simulink model "Target_Control_System"  (R2021b)
settings: Solver=FixedStepDiscrete  StartTime=0.0  StopTime=5  RelTol=1e-3
PreLoadFcn:
  | RTWConfigurationCB('preloadfcn', bdroot);
PostLoadFcn:
  | load('configuration/data_struct.mat');
  | load('configuration/fluxMaps_propMotor.mat');
  | load('configuration/parameterInit_PROP.mat');
  | load('configuration/parameterInit_PUMP.mat');
  | load('configuration/parameterInit_PITCH.mat');
  | load('configuration/parameterInit_TILT.mat');
  | %load('configuration/base_workspace_signal_definition.mat');
  | %load('resolvedatastores_to_baseworkspace_for_faster_simulation.mat');
model workspace (MAT data in the model file):
  SIMULATION_OPTIONS : Simulink.Parameter (value not decoded)
  TARGET_CODE_GEN : Simulink.Parameter (value not decoded)
  TCS_SAMPLE_FREQ_HZ : Simulink.Parameter (value not decoded)
symbols that are objects in the model workspace (value not decoded): TARGET_CODE_GEN, TCS_SAMPLE_FREQ_HZ
undefined symbols (not defined in the file): A_DQ_REF_LPF_INIT__PITCH, A_DQ_REF_LPF_INIT__PROP, A_DQ_REF_LPF_INIT__PUMP, A_DQ_REF_LPF_INIT__TILT, A_OBSERVER_CONFIDENCE_INIT__PITCH, A_OBSERVER_CONFIDENCE_INIT__PROP, A_OBSERVER_CONFIDENCE_INIT__PUMP, A_OBSERVER_CONFIDENCE_INIT__TILT, ACTUATOR_MAX_ANGLE_TRIP__PITCH, ACTUATOR_MIN_ANGLE_TRIP__PITCH, ACTUATOR_POS_SENSOR_INV_DIRECTION__PITCH, ACTUATOR_POS_SENSOR_INV_DIRECTION__TILT, ACTUATOR_POS_SENSOR_OFFSET__PITCH, ACTUATOR_POS_SENSOR_OFFSET__TILT, ADC_scaler1_baseaddr_TILT, ADC_SCALER_FLOAT_TO_FIXPOINT_EXPANSION, ANGLE_ELEC_FROM_SENSOR_OFFSET_INIT__PITCH, ANGLE_ELEC_FROM_SENSOR_OFFSET_INIT__PROP, ANGLE_ELEC_FROM_SENSOR_OFFSET_INIT__PUMP, ANGLE_ELEC_FROM_SENSOR_OFFSET_INIT__TILT, AUTO_CLEAR_FAULTS_ENABLED__PITCH, AUTO_CLEAR_FAULTS_ENABLED__PROP, AUTO_CLEAR_FAULTS_ENABLED__PUMP, AUTO_CLEAR_FAULTS_ENABLED__TILT, AUTO_CLEAR_FAULTS_WAIT_TICKS__PITCH, AUTO_CLEAR_FAULTS_WAIT_TICKS__PROP, AUTO_CLEAR_FAULTS_WAIT_TICKS__PUMP, AUTO_CLEAR_FAULTS_WAIT_TICKS__TILT, AUTO_I_ZERO_IDLE_TICKS__PITCH, AUTO_I_ZERO_IDLE_TICKS__PROP, AUTO_I_ZERO_IDLE_TICKS__PUMP, AUTO_I_ZERO_IDLE_TICKS__TILT, AUTO_I_ZERO_OFFSET_IDC_THRESHOLD__PITCH, AUTO_I_ZERO_OFFSET_IDC_THRESHOLD__PROP, AUTO_I_ZERO_OFFSET_IDC_THRESHOLD__PUMP, AUTO_I_ZERO_OFFSET_IDC_THRESHOLD__TILT, AUTO_I_ZERO_OFFSET_IPH_THRESHOLD__PITCH, AUTO_I_ZERO_OFFSET_IPH_THRESHOLD__PROP, AUTO_I_ZERO_OFFSET_IPH_THRESHOLD__PUMP, AUTO_I_ZERO_OFFSET_IPH_THRESHOLD__TILT, AUTO_SENSORLESS_SWITCHOVER_DISABLE_OMEGA, AUTO_SENSORLESS_SWITCHOVER_ENABLE_OMEGA, AUTO_SENSORLESS_SWITCHOVER_MIN_CONFIDENCE, AUXILIARY_PROTECTION_UNIT_BASEADDR__TILT, blanking_max_error_omega_INIT_PITCH, blanking_max_error_omega_INIT_TILT, blanking_max_error_position_INIT_PITCH, blanking_max_error_position_INIT_TILT, BRUTE_START_I_Q_REF_RAMP_SPEED__PITCH, BRUTE_START_I_Q_REF_RAMP_SPEED__PROP, BRUTE_START_I_Q_REF_RAMP_SPEED__PUMP, BRUTE_START_I_Q_REF_RAMP_SPEED__TILT, CONTROL_LOOP_DT_INIT__PITCH, CONTROL_LOOP_DT_INIT__PROP, CONTROL_LOOP_DT_INIT__PUMP, CONTROL_LOOP_DT_INIT__TILT, CORRECTION_FILTER_SCALE__PITCH, CORRECTION_FILTER_SCALE__PROP, CORRECTION_FILTER_SCALE__PUMP, CORRECTION_FILTER_SCALE__TILT ... (+458)
libraries: simulink x178, Reusables_Lib x24
(part 13 of 47)

== system Target_Control_System/Target_Control_System/InterruptFunction/tiltMotor_isrTask/pwmGeneration/Subsystem ==
  Enable : EnablePort
  ABC to DQ : Subsystem
  Calculate Duty Cycles : Subsystem
  Constant : Constant  OutDataTypeStr=int32  SampleTime=-1
  Constant1 : Constant  Commented=on  OutDataTypeStr=uint32  SampleTime=-1
  Data Store Read1 : DataStoreRead  DataStoreName=mdl_tilt_fFluxMasterAngleBkwd_cos_  IndexOptions=Index vector (dialog)  Indices=1  OutputSizes=1
  Data Store Read13 : DataStoreRead  DataStoreName=mdl_tilt_fFluxMasterAngleBkwd_sin_  IndexOptions=Index vector (dialog)  Indices=1  OutputSizes=1
  Data Store Read2 : DataStoreRead  DataStoreName=oTilt  DataStoreElements=oTilt.oIsr_.oParam_.iInverseDirection_  IndexOptions=Index vector (dialog)  Indices=1  OutputSizes=1
  Data Store Read3 : DataStoreRead  DataStoreName=oTilt  DataStoreElements=oTilt.oIsr_.oState_.fUdRef_  IndexOptions=Index vector (dialog)  Indices=1  OutputSizes=1
  Data Store Read4 : DataStoreRead  DataStoreName=oTilt  DataStoreElements=oTilt.oIsr_.oState_.fUqRef_  IndexOptions=Index vector (dialog)  Indices=1  OutputSizes=1
  Data Store Read6 : DataStoreRead  DataStoreName=oTilt  DataStoreElements=oTilt.oIsr_.oParam_.fMaximumDuty_  IndexOptions=Index vector (dialog)  Indices=1  OutputSizes=1
  Data Store Read7 : DataStoreRead  DataStoreName=oTilt  DataStoreElements=oTilt.oIsr_.oParam_.fHalfPositiveDuty_  IndexOptions=Index vector (dialog)  Indices=1  OutputSizes=1
  Data Store Read8 : DataStoreRead  DataStoreName=oTilt  DataStoreElements=oTilt.oIsr_.oParam_.fPwmPeriodTicksFloat_  IndexOptions=Index vector (dialog)  Indices=1  OutputSizes=1
  Data Store Write : DataStoreWrite  DataStoreName=oTilt  DataStoreElements=oTilt.oIsr_.oOut_.uiPwmDutyTicksA_  IndexOptions=Index vector (dialog)  Indices=1  OutputSizes=1
  Data Store Write1 : DataStoreWrite  DataStoreName=oTilt  DataStoreElements=oTilt.oIsr_.oOut_.uiPwmDutyTicksB_  IndexOptions=Index vector (dialog)  Indices=1  OutputSizes=1
  Data Store Write2 : DataStoreWrite  DataStoreName=oTilt  DataStoreElements=oTilt.oIsr_.oOut_.uiPwmDutyTicksC_  IndexOptions=Index vector (dialog)  Indices=1  OutputSizes=1
  Data Store Write3 : DataStoreWrite  Commented=on  DataStoreName=oTilt  DataStoreElements=oTilt.oIsr_.oOut_.uiPwmSetByIsr_  IndexOptions=Index vector (dialog)  Indices=1  OutputSizes=1
  Data Store Write4 : DataStoreWrite  DataStoreName=oTilt  DataStoreElements=oTilt.oIsr_.oState_.iPwmUpdated_  IndexOptions=Index vector (dialog)  Indices=1  OutputSizes=1
  Zero sequence injection : Subsystem
  wires:
  Constant1/1 -> Data Store Write3/1
  Data Store Read1/1 -> ABC to DQ/5(fFluxMasterAngleBkwd_cos)
  Data Store Read13/1 -> ABC to DQ/4(fFluxMasterAngleBkwd_sin)
  Calculate Duty Cycles/3(uiPwmDutyTicksC) -> Data Store Write2/1
  Calculate Duty Cycles/2(uiPwmDutyTicksB) -> Data Store Write1/1
  Calculate Duty Cycles/1(uiPwmDutyTicksA) -> Data Store Write/1
  Data Store Read3/1 -> ABC to DQ/2(UdRef)
  Data Store Read4/1 -> ABC to DQ/3(UqRef)
  Data Store Read8/1 -> Calculate Duty Cycles/6(fPwmPeriodTicksFloat)
  Data Store Read7/1 -> Calculate Duty Cycles/5(fHalfPositiveDuty)
  Data Store Read6/1 -> Calculate Duty Cycles/4(fMaximumDuty)
  Data Store Read2/1 -> ABC to DQ/1(iInverseDirection)
  Zero sequence injection/3(fUcRef) -> Calculate Duty Cycles/3(fUcRef)
  Zero sequence injection/2(fUbRef) -> Calculate Duty Cycles/2(fUbRef)
  Zero sequence injection/1(fUaRef) -> Calculate Duty Cycles/1(fUaRef)
  ABC to DQ/1(U_abc) -> Zero sequence injection/1(U_abc)
  Constant/1 -> Data Store Write4/1

== system Target_Control_System/Target_Control_System/InterruptFunction/tiltMotor_setPwm/ModelSourceFPGATilt/DoNotIncludeCustomCode ==

== system Target_Control_System/Target_Control_System/InterruptFunction/tiltMotor_setPwm/ModelSourceFPGATilt/IncludeCustomCode ==
  System Update : Subsystem  mask(System Update){ShowInLibBrowser=0}
      mask prompts: ShowInLibBrowser "Simulink:masks:CustCodeMaskParam1_MP"
      settings: CopyFcn=cccopyfcn(gcb)  OpenFcn=ccopenfcn('System Update Function')
      mask Help: eval('feval(''rtwprivate'',''rtwhelpview'',''rtw_sys_update_block'')');
      mask DialogControl ShowInLibBrowser Prompt: Mask Parameter 1:
      mask Display: disp('System\nUpdate');

== system Target_Control_System/Target_Control_System/MainLoop/pitchMotor_mainLoop/Decimation gate for 10 Hz Pitch/Function-Call Subsystem ==
  motorTaskMainDecimationBStep_pitch : TriggerPort  TriggerType=function-call  VariantControl=Variant
  DC_overvoltage_pitch : Stateflow chart  TreatAsAtomicUnit=on
  Dynamic_current_limiting_pitch : Subsystem

== system Target_Control_System/Target_Control_System/MainLoop/pitchMotor_mainLoop/Decimation gate for 200 Hz Pitch/Function-Call Subsystem ==
  motorTaskMainDecimationAStep_pitch : TriggerPort  TriggerType=function-call  VariantControl=Variant
  Check zero current if inverter off : Subsystem  TreatAsAtomicUnit=on
  Current control inactive : Subsystem  TreatAsAtomicUnit=on
  Current offset nulling : Subsystem  TreatAsAtomicUnit=on
  DClink_overCurrentProtection : Subsystem  TreatAsAtomicUnit=on
  Forced current injection for broken input sensors : Subsystem  Commented=on  TreatAsAtomicUnit=on
  Function-Call Generator : simulink/Ports & Subsystems/Function-Call Generator  sample_time=-1  numberOfIterations=1  DisallowWideOutput=off
  Function-Call Split{1..5,10} (6 alike) : FunctionCallSplit  NumOutputPorts=2
  Idle controller : Subsystem  TreatAsAtomicUnit=on
  Position control checks : Subsystem  TreatAsAtomicUnit=on
  wires:
  Function-Call Split10/2 -> Function-Call Split1/1
  Function-Call Split3/2 -> Function-Call Split4/1
  Function-Call Generator/1 -> Function-Call Split10/1
  Function-Call Split3/1 -> Current control inactive/Trigger
  Function-Call Split1/1 -> Check zero current if inverter off/Trigger
  Function-Call Split10/1 -> DClink_overCurrentProtection/Trigger
  Function-Call Split2/2 -> Function-Call Split3/1
  Function-Call Split5/1 -> Idle controller/Trigger
  Function-Call Split1/2 -> Function-Call Split2/1
  Function-Call Split4/1 -> Forced current injection for broken input sensors/Trigger
  Function-Call Split2/1 -> Current offset nulling/Trigger
  Function-Call Split5/2 -> Position control checks/Trigger
  Function-Call Split4/2 -> Function-Call Split5/1

== system Target_Control_System/Target_Control_System/MainLoop/pitchMotor_mainLoop/Decimation gate for 5000 Hz Pitch/motorTaskProcessExternalSetpoints(&oPitch) ==
  note: // Do not set certain variables during auto forced angle start or resistance measurement // This whole code below should be cleaned up, probably a switch case tied to the state machine.
      | // The different modes, (position control, speed control, current control) should get different state numbers to facilitate this.
  note: // Take externally requested setpoints (already set in the 'in' struct) and apply them (after sanitizing) to the right place in the control loop, also depending on the state that the drive is in.
  motorTaskProcessExternalSetpoints : TriggerPort  TriggerType=function-call  VariantControl=Variant
  Function-Call Generator : simulink/Ports & Subsystems/Function-Call Generator  sample_time=-1  numberOfIterations=1  DisallowWideOutput=off
  Function-Call Split1 : FunctionCallSplit  NumOutputPorts=2
  Function-Call Split10 : FunctionCallSplit  NumOutputPorts=2
  hot_standby : Subsystem
  passive_holding_mode : Subsystem
  set_target : Subsystem
  wires:
  Function-Call Split1/2 -> set_target/Trigger
  Function-Call Split10/2 -> Function-Call Split1/1
  Function-Call Split1/1 -> hot_standby/Trigger
  Function-Call Split10/1 -> passive_holding_mode/Trigger
  Function-Call Generator/1 -> Function-Call Split10/1

== system Target_Control_System/Target_Control_System/MainLoop/pitchMotor_mainLoop/mainTask_pitch/PWM for Simulation ==
  Enable : EnablePort
  Bus Creator3 : BusCreator  Inputs=3
  Constant : Constant  OutDataTypeStr=uint32  SampleTime=-1
  Constant{1..4} (4 alike) : Constant  Value=0  OutDataTypeStr=uint32  SampleTime=-1
  Data Store Read1 : DataStoreRead  DataStoreName=oPitch  DataStoreElements=oPitch.oIsr_.oState_.iPwmUpdated_  IndexOptions=Index vector (dialog)  Indices=1  OutputSizes=1
  Data Store Read9 : DataStoreRead  DataStoreName=oPitch  DataStoreElements=oPitch.oMot_.oOut_.uiEnableGateDrive_  IndexOptions=Index vector (dialog)  Indices=1  OutputSizes=1
  Data Store Write18 : DataStoreWrite  DataStoreName=oPitch  DataStoreElements=oPitch.oIsr_.oOut_.uiPwmSetByIsr_  IndexOptions=Index vector (dialog)  Indices=1  OutputSizes=1
  NOT : Logic  Operator=NOT  AllPortsSameDT=off  OutDataTypeStr=boolean
  Scope : Scope
  Subsystem : Subsystem
  Subsystem1 : Subsystem
  Switch1 : Switch  Criteria=u2 > Threshold
  Switch2 : Switch  Criteria=u2 > Threshold
  Switch3 : Switch  Criteria=u2 > Threshold
  Out1 : Outport
  wires:
  Switch3/1 -> Data Store Write18/1
  Constant4/1 -> Switch3/3
  Subsystem/1(pitchMotor_PWMticks) -> Switch2/1
  Constant/1 -> Switch3/1
  Subsystem1/1(pitchMotor_PWMticks) -> Switch2/3
  Data Store Read1/1 -> Subsystem/Enable, Switch2/2, NOT/1, Scope/1, Switch3/2
  NOT/1 -> Subsystem1/Enable
  Data Store Read9/1 -> Switch1/2
  Switch2/1 -> Switch1/1  "pitchMotor_PWMticks"
  Constant1/1 -> Bus Creator3/1  "Aticks"
  Constant2/1 -> Bus Creator3/2  "Bticks"
  Switch1/1 -> Out1/1  "pitchMotor_PWMticks"
  Constant3/1 -> Bus Creator3/3  "Cticks"
  Bus Creator3/1 -> Switch1/3

== system Target_Control_System/Target_Control_System/MainLoop/pitchMotor_mainLoop/mainTask_pitch/Variant Subsystem ==
  note: 1) Add Subsystem or Model blocks as valid variant choices.
      | 2) You cannot connect blocks at this level. At simulation, connectivity is automatically
      | determined, based on the active variant and port name matching.
  Target_Code_Gen_0 : Subsystem  VariantControl=(default)
  Target_Code_Gen_1 : Subsystem  VariantControl=TARGET_CODE_GEN==1
  Output : Outport  OutputFunctionCall=on

== system Target_Control_System/Target_Control_System/MainLoop/pitchMotor_mainLoop/mainTask_pitch/motorTaskMainFastStep() ==
  motorTaskMainFastStep : TriggerPort  TriggerType=function-call  VariantControl=Variant
  Automatic switching to sensorless - Pitch : Subsystem  Commented=on
  Control Loops - Pitch : Subsystem
  Correction Constants for Observer and Control - Pitch : Subsystem  Commented=on
  Function-Call Generator : simulink/Ports & Subsystems/Function-Call Generator  sample_time=-1  numberOfIterations=1  DisallowWideOutput=off
  Function-Call Split{1..6,10} (7 alike) : FunctionCallSplit  NumOutputPorts=2
  Lowpass Filtered Quantities for External World - Pitch : Subsystem
  Mechanical System - Pitch : Subsystem
  Motor Acceleration - Pitch : Subsystem
  Observer Confidence - Pitch : Subsystem  Commented=on
  Software Overcurrent Protection - Pitch : Subsystem
  enableDrive(&oPitch) : Stateflow chart  TreatAsAtomicUnit=on
  initiateOffsetNulling(&oPitch) : Stateflow chart  TreatAsAtomicUnit=on
  wires:
  Function-Call Split6/2 -> Motor Acceleration - Pitch/Trigger
  Function-Call Split6/1 -> Correction Constants for Observer and Control - Pitch/Trigger
  Function-Call Split5/2 -> Function-Call Split6/1
  Function-Call Split5/1 -> Control Loops - Pitch/Trigger
  Function-Call Split4/2 -> Function-Call Split5/1
  Function-Call Split4/1 -> Lowpass Filtered Quantities for External World - Pitch/Trigger
  Function-Call Split3/2 -> Function-Call Split4/1
  Function-Call Split3/1 -> Automatic switching to sensorless - Pitch/Trigger
  Function-Call Split2/2 -> Function-Call Split3/1
  Function-Call Split2/1 -> Observer Confidence - Pitch/Trigger
  Function-Call Split1/2 -> Function-Call Split2/1
  Function-Call Split1/1 -> Mechanical System - Pitch/Trigger
  Function-Call Generator/1 -> Function-Call Split10/1
  Function-Call Split10/1 -> Software Overcurrent Protection - Pitch/Trigger
  Function-Call Split10/2 -> Function-Call Split1/1

== system Target_Control_System/Target_Control_System/MainLoop/pitchMotor_mainLoop/mainTask_pitch/motorTaskManagePwmRequestFlags() ==
  motorTaskManagePwmRequestFlags : TriggerPort  TriggerType=function-call  VariantControl=Variant
  Constant : Constant  Value=0  OutDataTypeStr=uint32  SampleTime=-1
  Data Store Read : DataStoreRead  DataStoreName=oPitch  DataStoreElements=oPitch.oMot_.oIn_.uiPwmSetByIsr_  IndexOptions=Index vector (dialog)  Indices=1  OutputSizes=1
  Data Store Read1 : DataStoreRead  DataStoreName=oPitch  DataStoreElements=oPitch.oMot_.oOut_.uiPwmRequestFromMain_  IndexOptions=Index vector (dialog)  Indices=1  OutputSizes=1
  Data Store Write : DataStoreWrite  DataStoreName=oPitch  DataStoreElements=oPitch.oMot_.oOut_.uiPwmRequestFromMain_  IndexOptions=Index vector (dialog)  Indices=1  OutputSizes=1
  Switch : Switch  Criteria=u2 > Threshold  OutDataTypeStr=uint32
  wires:
  Data Store Read1/1 -> Switch/3
  Constant/1 -> Switch/1
  Switch/1 -> Data Store Write/1
  Data Store Read/1 -> Switch/2

== system Target_Control_System/Target_Control_System/MainLoop/pitchMotor_mainLoop/mainTask_pitch/resetFlag_uiDataFromIsrToMainUpdated ==
  resetFlag_uiDataFromIsrToMainUpdated : TriggerPort  TriggerType=function-call  VariantControl=Variant
  Constant : Constant  Value=0  OutDataTypeStr=uint32  SampleTime=-1
  Data Store Write : DataStoreWrite  DataStoreName=oPitch  DataStoreElements=oPitch.oMot_.oIn_.uiDataFromIsrToMainUpdated_  IndexOptions=Index vector (dialog)  Indices=1  OutputSizes=1
  wires:
  Constant/1 -> Data Store Write/1

== system Target_Control_System/Target_Control_System/MainLoop/propMotor_mainLoop/Decimation gate A for 200 Hz Prop/Cross-tripping VP//Tilt to Prop ==
  Tilt to Prop : Stateflow chart  TreatAsAtomicUnit=on
  VP to Prop : Stateflow chart  TreatAsAtomicUnit=on

== system Target_Control_System/Target_Control_System/MainLoop/propMotor_mainLoop/Decimation gate A for 200 Hz Prop/Current offset nulling ==
  note: Try to perform current sensor offset nulling at least once as soon as possible:
      | (Subsequent nulling steps are performed only once the drive has been idle for a while)
  function : TriggerPort  TriggerType=function-call  VariantControl=Variant
  Constant2 : Constant  Value=0  OutDataTypeStr=uint32  SampleTime=-1
  Data Store Read2 : DataStoreRead  DataStoreName=oProp  DataStoreElements=oProp.oMot_.oState_.uiCurrentOffsetNullingPerformed_  IndexOptions=Index vector (dialog)  Indices=1  OutputSizes=1
  GreaterThan1 : RelationalOperator  Operator=>  OutDataTypeStr=boolean  RndMeth=Simplest
  NOT : Logic  Operator=NOT  IconShape=distinctive  AllPortsSameDT=off  OutDataTypeStr=boolean
  initiateOffsetNulling(&oProp) : Subsystem  TreatAsAtomicUnit=on
  wires:
  NOT/1 -> initiateOffsetNulling(&oProp)/Enable
  GreaterThan1/1 -> NOT/1
  Constant2/1 -> GreaterThan1/2
  Data Store Read2/1 -> GreaterThan1/1

== system Target_Control_System/Target_Control_System/MainLoop/propMotor_mainLoop/Decimation gate A for 200 Hz Prop/Subsystem ==
  Idle_Controller : TriggerPort  TriggerType=function-call  VariantControl=Variant
  AND7 : Logic  AllPortsSameDT=off  OutDataTypeStr=boolean
  Data Store Read1 : DataStoreRead  DataStoreName=oProp  DataStoreElements=oProp.oMot_.oParam_.oPiDataIdleCtrl_.fState_  IndexOptions=Index vector (dialog)  Indices=1  OutputSizes=1
  Data Store Read12 : DataStoreRead  DataStoreName=oProp  DataStoreElements=oProp.oMot_.oState_.uiDriveState_  IndexOptions=Index vector (dialog)  Indices=1  OutputSizes=1
  Data Store Read2 : DataStoreRead  DataStoreName=oProp  DataStoreElements=oProp.oMot_.oParam_.fRpmBlankingUnblankConfidence_  IndexOptions=Index vector (dialog)  Indices=1  OutputSizes=1
  Data Store Read3 : DataStoreRead  DataStoreName=oProp  DataStoreElements=oProp.oMot_.oParam_.fRpmBlankingBlankConfidence_  IndexOptions=Index vector (dialog)  Indices=1  OutputSizes=1
  Data Store Read51 : DataStoreRead  DataStoreName=oProp  DataStoreElements=oProp.oMot_.oState_.uiDriveState_  IndexOptions=Index vector (dialog)  Indices=1  OutputSizes=1
  Data Store Read65 : DataStoreRead  DataStoreName=oProp  DataStoreElements=oProp.oMot_.oOut_.fOmegaEObserverXlpf2_  IndexOptions=Index vector (dialog)  Indices=1  OutputSizes=1
  Data Store Read66 : DataStoreRead  DataStoreName=oProp  DataStoreElements=oProp.oMot_.oState_.fIdleCtrlOmegaEMin_  IndexOptions=Index vector (dialog)  Indices=1  OutputSizes=1
  Data Store Read67 : DataStoreRead  DataStoreName=oProp  DataStoreElements=oProp.oMot_.oParam_.oPiDataIdleCtrl_.oParameter_.fKp_  IndexOptions=Index vector (dialog)  Indices=1  OutputSizes=1
  Data Store Read69 : DataStoreRead  DataStoreName=oProp  DataStoreElements=oProp.oMot_.oParam_.oPiDataIdleCtrl_.oParameter_.fKi_  IndexOptions=Index vector (dialog)  Indices=1  OutputSizes=1
  Data Store Read70 : DataStoreRead  DataStoreName=oProp  DataStoreElements=oProp.oMot_.oParam_.oPiDataIdleCtrl_.oParameter_.fIntMax_  IndexOptions=Index vector (dialog)  Indices=1  OutputSizes=1
  Data Store Read80 : DataStoreRead  DataStoreName=oProp  DataStoreElements=oProp.oMot_.oState_.fObserverConfidence_  IndexOptions=Index vector (dialog)  Indices=1  OutputSizes=1
  Data Store Read94 : DataStoreRead  DataStoreName=oProp  DataStoreElements=oProp.oMot_.oParam_.oPiDataIdleCtrl_.oParameter_.fOutMax_  IndexOptions=Index vector (dialog)  Indices=1  OutputSizes=1
  Data Store Read95 : DataStoreRead  DataStoreName=oProp  DataStoreElements=oProp.oMot_.oParam_.oPiDataIdleCtrl_.oParameter_.fLoopDt_  IndexOptions=Index vector (dialog)  Indices=1  OutputSizes=1
  Data Store Write10 : DataStoreWrite  DataStoreName=oProp  DataStoreElements=oProp.oMot_.oState_.iRpmBlankingActive_  IndexOptions=Index vector (dialog)  Indices=1  OutputSizes=1
  Equal12 : RelationalOperator  Operator===  OutDataTypeStr=boolean  RndMeth=Simplest
  Equal16 : RelationalOperator  Operator=~=  OutDataTypeStr=boolean  RndMeth=Simplest
  Equal17 : RelationalOperator  Operator=~=  OutDataTypeStr=boolean  RndMeth=Simplest
  NOT : Logic  Operator=NOT  AllPortsSameDT=off  OutDataTypeStr=boolean
  OR (Never blank in state 200)1 : Logic  Operator=OR  AllPortsSameDT=off  OutDataTypeStr=boolean
  Subsystem : Subsystem
  Switch7 : Switch  Criteria=u2 > Threshold  Threshold=0.5  OutDataTypeStr=int32
  Zero18 : Constant  Value=0  OutDataTypeStr=single  SampleTime=-1
  Zero19 : Constant  OutDataTypeStr=single  SampleTime=-1
  Zero9 : Constant  Value=0  OutDataTypeStr=single  SampleTime=-1
  const12 : Constant  Value=200  OutDataTypeStr=uint32  SampleTime=-1
  const13 : Constant  Value=211  OutDataTypeStr=uint32  SampleTime=-1
  const14 : Constant  Value=212  OutDataTypeStr=uint32  SampleTime=-1
  greater1 : RelationalOperator  Operator=>  OutDataTypeStr=boolean  RndMeth=Simplest
  piControllerStep_Idle_Controller : Subsystem  SystemSampleTime=1/200
  smaller1 : RelationalOperator  Operator=<  OutDataTypeStr=boolean  RndMeth=Simplest
  wires:
  Data Store Read80/1 -> smaller1/1, greater1/1
  OR (Never blank in state 200)1/1 -> Switch7/2
  Zero9/1 -> Switch7/1
  smaller1/1 -> Switch7/3
  Equal12/1 -> OR (Never blank in state 200)1/1
  Data Store Read12/1 -> Equal12/1
  Data Store Read3/1 -> smaller1/2
  Data Store Read2/1 -> greater1/2
  Switch7/1 -> Data Store Write10/1
  const12/1 -> Equal12/2
  greater1/1 -> OR (Never blank in state 200)1/2
  NOT/1 -> Subsystem/Enable
  Data Store Read1/1 -> piControllerStep_Idle_Controller/11(fState)
  const13/1 -> Equal16/1
  Data Store Read67/1 -> piControllerStep_Idle_Controller/3(fKp)
  Data Store Read94/1 -> piControllerStep_Idle_Controller/8(fOutMax)
  Data Store Read66/1 -> piControllerStep_Idle_Controller/2(fTarget)
  Zero19/1 -> piControllerStep_Idle_Controller/5(fScale)
  Data Store Read70/1 -> piControllerStep_Idle_Controller/7(fIntMax)
  Data Store Read95/1 -> piControllerStep_Idle_Controller/6(fLoopDt)
  Data Store Read69/1 -> piControllerStep_Idle_Controller/4(fKi)
  Data Store Read51/1 -> Equal16/2, Equal17/1
  Equal17/1 -> AND7/2
  Zero18/1 -> piControllerStep_Idle_Controller/9(fIntMin), piControllerStep_Idle_Controller/10(fOutMin)
  AND7/1 -> piControllerStep_Idle_Controller/Enable, NOT/1
  const14/1 -> Equal17/2
  Data Store Read65/1 -> piControllerStep_Idle_Controller/1(fActual)
  Equal16/1 -> AND7/1

== system Target_Control_System/Target_Control_System/MainLoop/propMotor_mainLoop/Decimation gate for 5000 Hz Prop/motorTaskProcessExternalSetpoints(&oProp) ==
  note: // Do not set certain variables during auto forced angle start or resistance measurement // This whole code below should be cleaned up, probably a switch case tied to the state machine.
      | // The different modes, (position control, speed control, current control) should get different state numbers to facilitate this.
  note: // Take externally requested setpoints (already set in the 'in' struct) and apply them (after sanitizing) to the right place in the control loop, also depending on the state that the drive is in.
  motorTaskProcessExternalSetpoints : TriggerPort  TriggerType=function-call  VariantControl=Variant
  Function-Call Generator : simulink/Ports & Subsystems/Function-Call Generator  sample_time=-1  numberOfIterations=1  DisallowWideOutput=off
  Function-Call Split1 : FunctionCallSplit  NumOutputPorts=2
  Function-Call Split10 : FunctionCallSplit  NumOutputPorts=2
  Subsystem1 : Subsystem
  Subsystem2 : Subsystem
  Subsystem3 : Subsystem
  wires:
  Function-Call Split1/2 -> Subsystem3/Trigger
  Function-Call Split10/2 -> Function-Call Split1/1
  Function-Call Split1/1 -> Subsystem2/Trigger
  Function-Call Split10/1 -> Subsystem1/Trigger
  Function-Call Generator/1 -> Function-Call Split10/1

== system Target_Control_System/Target_Control_System/MainLoop/propMotor_mainLoop/motorTaskMainFastStep(&oProp)/Control Loops - Prop ==
  note: ---------- runFluxWeakeningCurrentCalculation ------------
      | 	// This function calculates how much flux weakening current is needed to keep the modulation index below full scale.
      | 	// It uses positive numbers exclusively for ease of reading & reasoning; the calling function
      | 	// will have to include a minus sign somewhere to turn it into negative d-current.
  note: // If the speed is too low, just return zero. // This is a simple safety catch to prevent injecting d current when there should be no need for it.
  note: mdl_fIdFluxWeakeningSetpoint_
  controlLoops : TriggerPort  TriggerType=function-call  VariantControl=Variant
  AND1 : Logic  AllPortsSameDT=off  OutDataTypeStr=boolean
  Abs6 : Abs
  Add12 : Sum  Inputs=+-
  Constant3 : Constant  Value=0  OutDataTypeStr=single  SampleTime=-1
  Data Store Read1 : DataStoreRead  DataStoreName=oProp  DataStoreElements=oProp.oMot_.oState_.oRampDataFluxMstrAngFrcd2clsdSmoothn_.oParam_.fTimestepS_  IndexOptions=Index vector (dialog)  Indices=1  OutputSizes=1
  Data Store Read10 : DataStoreRead  Commented=on  DataStoreName=oProp  DataStoreElements=oProp.oMot_.oState_.oRampDataOmegaERef_.oParam_.fUpslope_  IndexOptions=Index vector (dialog)  Indices=1  OutputSizes=1
  Data Store Read100 : DataStoreRead  Commented=on  DataStoreName=oProp  DataStoreElements=oProp.oMot_.oState_.fForcedAngleStartOrigOmegaRamp_  IndexOptions=Index vector (dialog)  Indices=1  OutputSizes=1
  Data Store Read104 : DataStoreRead  Commented=on  DataStoreName=oProp  DataStoreElements=oProp.oMot_.oState_.fForcedAngleStartOrigIRamp_  IndexOptions=Index vector (dialog)  Indices=1  OutputSizes=1
  Data Store Read105 : DataStoreRead  Commented=on  DataStoreName=oProp  DataStoreElements=oProp.oMot_.oState_.oRampDataIqRef_.oParam_.fUpslope_  IndexOptions=Index vector (dialog)  Indices=1  OutputSizes=1
  Data Store Read106 : DataStoreRead  Commented=on  DataStoreName=oProp  DataStoreElements=oProp.oMot_.oParam_.fForcedAngleOmegaEHandoff_  IndexOptions=Index vector (dialog)  Indices=1  OutputSizes=1
  Data Store Read11 : DataStoreRead  Commented=on  DataStoreName=oProp  DataStoreElements=oProp.oMot_.oState_.oRampDataFluxMstrAngFrcd2clsdSmoothn_.oParam_.fUpslope_  IndexOptions=Index vector (dialog)  Indices=1  OutputSizes=1
  Data Store Read13 : DataStoreRead  Commented=on  DataStoreName=oProp  DataStoreElements=oProp.oMot_.oState_.oRampDataFluxMstrAngFrcd2clsdSmoothn_.oParam_.fDownslope_  IndexOptions=Index vector (dialog)  Indices=1  OutputSizes=1
  Data Store Read15 : DataStoreRead  DataStoreName=oProp  DataStoreElements=oProp.oMot_.oState_.oRampDataFluxMasterAngleOffset_.oParam_.fUpslope_  IndexOptions=Index vector (dialog)  Indices=1  OutputSizes=1
  Data Store Read16 : DataStoreRead  Commented=on  DataStoreName=oProp  DataStoreElements=oProp.oMot_.oState_.oRampDataFluxMstrAngFrcd2clsdSmoothn_.fRampOut_  IndexOptions=Index vector (dialog)  Indices=1  OutputSizes=1
  Data Store Read2 : DataStoreRead  DataStoreName=oProp  DataStoreElements=oProp.oMot_.oState_.oRampDataFluxMstrAngFrcd2clsdSmoothn_.oParam_.fUpslope_  IndexOptions=Index vector (dialog)  Indices=1  OutputSizes=1
  Data Store Read3 : DataStoreRead  DataStoreName=oProp  DataStoreElements=oProp.oMot_.oState_.oRampDataFluxMstrAngFrcd2clsdSmoothn_.oParam_.fDownslope_  IndexOptions=Index vector (dialog)  Indices=1  OutputSizes=1
  Data Store Read31 : DataStoreRead  DataStoreName=oProp  DataStoreElements=oProp.oMot_.oIn_.fOmegaEObserverLpf2_  IndexOptions=Index vector (dialog)  Indices=1  OutputSizes=1
  Data Store Read34 : DataStoreRead  DataStoreName=oProp  DataStoreElements=oProp.oMot_.oParam_.fIqSetpointMax_  IndexOptions=Index vector (dialog)  Indices=1  OutputSizes=1
  Data Store Read35 : DataStoreRead  DataStoreName=oProp  DataStoreElements=oProp.oMot_.oParam_.fDynILimIntegratorLeakageFactor_  IndexOptions=Index vector (dialog)  Indices=1  OutputSizes=1
  Data Store Read36 : DataStoreRead  DataStoreName=oProp  DataStoreElements=oProp.oMot_.oState_.fIqRefBeforeRamp_  IndexOptions=Index vector (dialog)  Indices=1  OutputSizes=1
  Data Store Read38 : DataStoreRead  DataStoreName=oProp  DataStoreElements=oProp.oMot_.oState_.fIdleCtrlCurrent_  IndexOptions=Index vector (dialog)  Indices=1  OutputSizes=1
  Data Store Read4 : DataStoreRead  DataStoreName=oProp  DataStoreElements=oProp.oMot_.oState_.oRampDataFluxMasterAngleOffset_.fSetpoint_  IndexOptions=Index vector (dialog)  Indices=1  OutputSizes=1
  Data Store Read5 : DataStoreRead  DataStoreName=oProp  DataStoreElements=oProp.oMot_.oState_.oRampDataIqRef_.fRampOut_  IndexOptions=Index vector (dialog)  Indices=1  OutputSizes=1
  Data Store Read63 : DataStoreRead  DataStoreName=oProp  DataStoreElements=oProp.oMot_.oState_.oRampDataFluxMasterAngleOffset_.oParam_.fDownslope_  IndexOptions=Index vector (dialog)  Indices=1  OutputSizes=1
  Data Store Read64 : DataStoreRead  DataStoreName=oProp  DataStoreElements=oProp.oMot_.oState_.oRampDataFluxMasterAngleOffset_.oParam_.fTimestepS_  IndexOptions=Index vector (dialog)  Indices=1  OutputSizes=1
  Data Store Read65 : DataStoreRead  DataStoreName=oProp  DataStoreElements=oProp.oMot_.oParam_.fFluxWeakeningMinimumOmegaE_  IndexOptions=Index vector (dialog)  Indices=1  OutputSizes=1
  Data Store Read71 : DataStoreRead  DataStoreName=oProp  DataStoreElements=oProp.oMot_.oState_.oRampDataIqRef_.oParam_.fTimestepS_  IndexOptions=Index vector (dialog)  Indices=1  OutputSizes=1
  Data Store Read73 : DataStoreRead  DataStoreName=oProp  DataStoreElements=oProp.oMot_.oState_.oRampDataIqRef_.oParam_.fUpslope_  IndexOptions=Index vector (dialog)  Indices=1  OutputSizes=1
  Data Store Read76 : DataStoreRead  DataStoreName=oProp  DataStoreElements=oProp.oMot_.oState_.oRampDataIqRef_.oParam_.fDownslope_  IndexOptions=Index vector (dialog)  Indices=1  OutputSizes=1
  Data Store Read77 : DataStoreRead  DataStoreName=oProp  DataStoreElements=oProp.oMot_.oState_.oRampDataOmegaERef_.oParam_.fTimestepS_  IndexOptions=Index vector (dialog)  Indices=1  OutputSizes=1
  Data Store Read78 : DataStoreRead  DataStoreName=oProp  DataStoreElements=oProp.oMot_.oState_.oRampDataOmegaERef_.oParam_.fUpslope_  IndexOptions=Index vector (dialog)  Indices=1  OutputSizes=1
  Data Store Read81 : DataStoreRead  DataStoreName=oProp  DataStoreElements=oProp.oMot_.oState_.oRampDataIdRef_.oParam_.fTimestepS_  IndexOptions=Index vector (dialog)  Indices=1  OutputSizes=1
  Data Store Read82 : DataStoreRead  DataStoreName=oProp  DataStoreElements=oProp.oMot_.oState_.oRampDataOmegaERef_.fSetpoint_  IndexOptions=Index vector (dialog)  Indices=1  OutputSizes=1
  Data Store Read84 : DataStoreRead  DataStoreName=oProp  DataStoreElements=oProp.oMot_.oState_.oRampDataIdRef_.oParam_.fUpslope_  IndexOptions=Index vector (dialog)  Indices=1  OutputSizes=1
  Data Store Read85 : DataStoreRead  DataStoreName=oProp  DataStoreElements=oProp.oMot_.oState_.oRampDataIdRef_.oParam_.fDownslope_  IndexOptions=Index vector (dialog)  Indices=1  OutputSizes=1
  Data Store Read87 : DataStoreRead  DataStoreName=oProp  DataStoreElements=oProp.oMot_.oState_.oRampDataOmegaERef_.oParam_.fDownslope_  IndexOptions=Index vector (dialog)  Indices=1  OutputSizes=1
  Data Store Read88 : DataStoreRead  DataStoreName=oProp  DataStoreElements=oProp.oMot_.oState_.fIdExternalSetpoint_  IndexOptions=Index vector (dialog)  Indices=1  OutputSizes=1
  Data Store Write1 : DataStoreWrite  Commented=on  DataStoreName=oProp  DataStoreElements=oProp.oMot_.oState_.oRampDataFluxMstrAngFrcd2clsdSmoothn_.fRampOut_  IndexOptions=Index vector (dialog)  Indices=1  OutputSizes=1
  Data Store Write14 : DataStoreWrite  DataStoreName=oProp  DataStoreElements=oProp.oMot_.oState_.oRampDataIdRef_.fRampOut_  IndexOptions=Index vector (dialog)  Indices=1  OutputSizes=1
  Data Store Write15 : DataStoreWrite  DataStoreName=oProp  DataStoreElements=oProp.oMot_.oState_.oRampDataIdRef_.fRampOutDdt_  IndexOptions=Index vector (dialog)  Indices=1  OutputSizes=1
  Data Store Write18 : DataStoreWrite  DataStoreName=oProp  DataStoreElements=oProp.oMot_.oState_.oRampDataIqRef_.fRampOut_  IndexOptions=Index vector (dialog)  Indices=1  OutputSizes=1
  Data Store Write19 : DataStoreWrite  DataStoreName=oProp  DataStoreElements=oProp.oMot_.oState_.oRampDataIqRef_.fSetpoint_  IndexOptions=Index vector (dialog)  Indices=1  OutputSizes=1
  Data Store Write2 : DataStoreWrite  DataStoreName=oProp  DataStoreElements=oProp.oMot_.oState_.oRampDataFluxMstrAngFrcd2clsdSmoothn_.fRampOut_  IndexOptions=Index vector (dialog)  Indices=1  OutputSizes=1
  Data Store Write23 : DataStoreWrite  DataStoreName=oProp  DataStoreElements=oProp.oMot_.oState_.oRampDataOmegaERef_.fRampOut_  IndexOptions=Index vector (dialog)  Indices=1  OutputSizes=1
  Data Store Write26 : DataStoreWrite  DataStoreName=oProp  DataStoreElements=oProp.oMot_.oState_.oRampDataIqRef_.fRampOutDdt_  IndexOptions=Index vector (dialog)  Indices=1  OutputSizes=1
  Data Store Write27 : DataStoreWrite  DataStoreName=oProp  DataStoreElements=oProp.oMot_.oState_.oRampDataOmegaERef_.fRampOutDdt_  IndexOptions=Index vector (dialog)  Indices=1  OutputSizes=1
  Data Store Write3 : DataStoreWrite  DataStoreName=oProp  DataStoreElements=oProp.oMot_.oState_.oRampDataFluxMstrAngFrcd2clsdSmoothn_.fRampOutDdt_  IndexOptions=Index vector (dialog)  Indices=1  OutputSizes=1
  Data Store Write35 : DataStoreWrite  DataStoreName=oProp  DataStoreElements=oProp.oMot_.oState_.oRampDataFluxMasterAngleOffset_.fRampOut_  IndexOptions=Index vector (dialog)  Indices=1  OutputSizes=1
  Data Store Write4 : DataStoreWrite  DataStoreName=oProp  DataStoreElements=oProp.oMot_.oState_.oRampDataFluxMstrAngFrcd2clsdSmoothn_.fSetpoint_  IndexOptions=Index vector (dialog)  Indices=1  OutputSizes=1
  Data Store Write44 : DataStoreWrite  DataStoreName=oProp  DataStoreElements=oProp.oMot_.oState_.oRampDataFluxMasterAngleOffset_.fRampOutDdt_  IndexOptions=Index vector (dialog)  Indices=1  OutputSizes=1
  Data Store Write7 : DataStoreWrite  DataStoreName=oProp  DataStoreElements=oProp.oMot_.oState_.oRampDataIdRef_.fSetpoint_  IndexOptions=Index vector (dialog)  Indices=1  OutputSizes=1
  Data Store Write9 : DataStoreWrite  DataStoreName=oProp  DataStoreElements=oProp.oMot_.oState_.fFluxWeakeningState_  IndexOptions=Index vector (dialog)  Indices=1  OutputSizes=1
  Dynamic Current Limiting Prop : Subsystem  TreatAsAtomicUnit=on
  Equal1 : RelationalOperator  Operator=>  OutDataTypeStr=boolean  RndMeth=Simplest
  Equal2 : RelationalOperator  Operator=>  OutDataTypeStr=boolean  RndMeth=Simplest
  Equal3 : RelationalOperator  Operator=<  OutDataTypeStr=boolean  RndMeth=Simplest
  Gain3 : Gain  Commented=on  Gain=-1
  Gain4 : Gain  Gain=-1
  Max1 : MinMax  Function=max  Inputs=2
  Min : MinMax  Inputs=2
  NOT1 : Logic  Operator=NOT  AllPortsSameDT=off  OutDataTypeStr=boolean
  Rate Limiter Dynamic1 : simulink/Discontinuities/Rate Limiter Dynamic  Commented=on
  Scope : Scope  Commented=on  NumInputPorts=3
  Scope1 : Scope  Commented=on  NumInputPorts=2
  Sim Options Prop Id Variant Subsystem : Subsystem  Variant=on
  Sim Options Prop Iq Variant Subsystem : Subsystem  Variant=on
  Subsystem2 : Subsystem
  Switch5 : Switch  Criteria=u2 > Threshold  Threshold=0.5
  Switch6 : Switch  Criteria=u2 > Threshold  Threshold=0.5
  Switch8 : Switch  Criteria=u2 > Threshold
  Zero1 : Constant  Value=0.001  OutDataTypeStr=single  SampleTime=-1
  Zero11 : Constant  Value=0  OutDataTypeStr=single  SampleTime=-1
  rampStep_oRampDataFluxMasterAngleOffset_ : Reusables_Lib/rampStep_  SystemSampleTime=-1  VariantActivationTime=update diagram  Latency=0  AutoFrameSizeCalculation=off
  rampStep_oRampDataFluxMstrAngFrcd2clsdSmoothn_ : Reusables_Lib/rampStep_  SystemSampleTime=-1  VariantActivationTime=update diagram  Latency=0  AutoFrameSizeCalculation=off
  rampStep_oRampDataIdRef_ : Reusables_Lib/rampStep_  SystemSampleTime=-1  VariantActivationTime=update diagram  Latency=0  AutoFrameSizeCalculation=off
  rampStep_oRampDataIqRef_ : Subsystem  AncestorBlock=Reusables_Lib/rampStep_
  rampStep_oRampDataOmegaERef_ : Reusables_Lib/rampStep_  SystemSampleTime=-1  VariantActivationTime=update diagram  Latency=0  AutoFrameSizeCalculation=off
  wires:
  Data Store Read5/1 -> rampStep_oRampDataIqRef_/5(fRampOut_z)
  rampStep_oRampDataFluxMasterAngleOffset_/2 -> Data Store Write44/1
  Data Store Read1/1 -> rampStep_oRampDataFluxMstrAngFrcd2clsdSmoothn_/4
  rampStep_oRampDataFluxMstrAngFrcd2clsdSmoothn_/1 -> Data Store Write2/1
  Data Store Read4/1 -> rampStep_oRampDataFluxMasterAngleOffset_/1
  Data Store Read63/1 -> rampStep_oRampDataFluxMasterAngleOffset_/3
  Data Store Read2/1 -> rampStep_oRampDataFluxMstrAngFrcd2clsdSmoothn_/2
  Data Store Read3/1 -> rampStep_oRampDataFluxMstrAngFrcd2clsdSmoothn_/3
  rampStep_oRampDataFluxMasterAngleOffset_/1 -> Data Store Write35/1
  rampStep_oRampDataFluxMstrAngFrcd2clsdSmoothn_/2 -> Data Store Write3/1
  Zero11/1 -> Data Store Write4/1, rampStep_oRampDataFluxMstrAngFrcd2clsdSmoothn_/1
  Data Store Read64/1 -> rampStep_oRampDataFluxMasterAngleOffset_/4
  Data Store Read15/1 -> rampStep_oRampDataFluxMasterAngleOffset_/2
  Subsystem2/1(Out1) -> Switch5/3, Data Store Write9/1
  Data Store Read65/1 -> Equal3/2
  Data Store Read31/1 -> Abs6/1
  Equal3/1 -> Switch5/2, NOT1/1
  NOT1/1 -> Subsystem2/Enable
  Data Store Read88/1 -> Add12/1
  Abs6/1 -> Equal3/1
  Constant3/1 -> Switch5/1
  Add12/1 -> Data Store Write7/1
  Switch5/1 -> Add12/2
  rampStep_oRampDataOmegaERef_/2 -> Data Store Write27/1
  Data Store Read11/1 -> Rate Limiter Dynamic1/1
  Data Store Read38/1 -> Switch6/1, Equal1/1, Equal2/1
  Data Store Read16/1 -> Rate Limiter Dynamic1/2
  Data Store Read34/1 -> Gain4/1, Min/2
  Switch6/1 -> Data Store Write19/1  "fIdleCtrlCurrent_"
  Equal2/1 -> AND1/2
  Data Store Read10/1 -> Scope/1
  Sim Options Prop Id Variant Subsystem/1(Out1) -> rampStep_oRampDataIdRef_/1
  AND1/1 -> Switch6/2
  Data Store Read87/1 -> rampStep_oRampDataOmegaERef_/3
  Data Store Read82/1 -> rampStep_oRampDataOmegaERef_/1
  rampStep_oRampDataIdRef_/1 -> Data Store Write14/1
  Data Store Read73/1 -> rampStep_oRampDataIqRef_/2(fUpslope_)
  Sim Options Prop Iq Variant Subsystem/1(Out1) -> rampStep_oRampDataIqRef_/1(fSetpoint_)
  Gain3/1 -> Rate Limiter Dynamic1/3
  rampStep_oRampDataIdRef_/2 -> Data Store Write15/1
  Data Store Read35/1 -> Dynamic Current Limiting Prop/Enable, Switch8/2
  Data Store Read76/1 -> rampStep_oRampDataIqRef_/3(fDDownslope_)
  Data Store Read36/1 -> Min/1
  Max1/1 -> Switch8/3
  Min/1 -> Max1/1
  Data Store Read78/1 -> rampStep_oRampDataOmegaERef_/2
  Data Store Read105/1 -> Scope1/2
  Gain4/1 -> Max1/2
  Data Store Read106/1 -> Scope/3
  Data Store Read84/1 -> rampStep_oRampDataIdRef_/2
  rampStep_oRampDataIqRef_/1(fRampOut_) -> Data Store Write18/1
  Data Store Read13/1 -> Gain3/1
  Data Store Read85/1 -> rampStep_oRampDataIdRef_/3
  Equal1/1 -> AND1/1
  Dynamic Current Limiting Prop/1(oRampDataIqRef_.fSetpoint) -> Switch8/1
  Data Store Read81/1 -> rampStep_oRampDataIdRef_/4
  Data Store Read104/1 -> Scope1/1
  Data Store Read77/1 -> rampStep_oRampDataOmegaERef_/4
  Data Store Read71/1 -> rampStep_oRampDataIqRef_/4(fTimestepS_)
  rampStep_oRampDataOmegaERef_/1 -> Data Store Write23/1
  Switch8/1 -> Equal2/2, Switch6/3
  Zero1/1 -> Equal1/2
  rampStep_oRampDataIqRef_/2(fRampOutDdt_) -> Data Store Write26/1
  Rate Limiter Dynamic1/1 -> Data Store Write1/1
  Data Store Read100/1 -> Scope/2

== system Target_Control_System/Target_Control_System/MainLoop/propMotor_mainLoop/motorTaskMainFastStep(&oProp)/Correction Constants for Observer and Control - Prop ==
  note: // ---------------- Correction constants for observer and control ------------
      | 	// Sources of delay:
      | 	//  1. Input.
      | 	//     a) delays from ADCs. Both voltage and current channels use identical ADCs and
      | 	//        initial FPGA processing. The delay on the current channel is taken as a
      | 	//        baseline.
      | 	//
      | 	//     b) Extra delays in the voltage acquisition stage, due to
      | 	//      1) tighter analog filtering
      | 	//      2) the 2 pole LPF filter in the FPGA.
      | 	//
      | 	//  2. Output
      | 	//     a) The PWM duty is updated only once per cycle, causing some delay.
      | 	//        Additionally, the interrupt might be delayed, causing further delays.
      | 	//
      | 	//  3. User specified for testing
      | 	//
      | 	// Values of the above delays:
      | 	//   1.a    A known constant delay is specified for each motor channel. (Mostly driven by the sinc3 filtering.
      |       //            Directly depends on sigma delta frequency.)
      | 	//   1.b.1  A known constant delay is specified for each motor channel
      | 	//   1.b.2  Can be calculated analytically
      | 	//   2.a    Approximated as a constant fraction of the PWM period.
      | 	//
      | 	// Compensation order of the above delays
      | 	//  - The entire interrupt loop runs behind reality by amount 1.a
      | 	//  - The delay on the current acquisition is therefore not compensated at the input to the algorithm.
      | 	//  - The voltage feedback needs to be aligned with the current feedback, and therefore needs to be
      | 	//    corrected for delays 1.b.1 and 1.b.2. This is a phase shift applied to the voltage.
      | 	//  - After the control loop, when the dq quantities are transformed to abc, the remaining delays are
      | 	//    corrected by phase shifting the dq angle. These delays are 1.a, 2.a and 3.
      | 	//
      | 	// Additionally, filter 1.b.2 causes a reduction in amplitude. This is compensated too to ensure
      | 	// a more level flux estimate output at high speeds.
      | 	//
  correctionConstantsObserverControl : TriggerPort  TriggerType=function-call  VariantControl=Variant
  Abs : Abs  OutDataTypeStr=single
  Abs1 : Abs  OutDataTypeStr=single
  Abs4 : Abs  OutDataTypeStr=single
  Add4 : Sum  Inputs=|++
  Add5 : Sum
  AmplitudeRatio : Fcn  Expr=1/sqrt(1+(u*u))
  Atan3 : Trigonometry  Operator=atan2
  Data Store Read14 : DataStoreRead  DataStoreName=oProp  DataStoreElements=oProp.oMot_.oParam_.fIntControlLoopDt_  IndexOptions=Index vector (dialog)  Indices=1  OutputSizes=1
  Data Store Read26 : DataStoreRead  DataStoreName=mdl_prop_fOmegaE  IndexOptions=Index vector (dialog)  Indices=1  OutputSizes=1
  Data Store Read33 : DataStoreRead  DataStoreName=oProp  DataStoreElements=oProp.oMot_.oParam_.fHardwareDelayVoltageAcquisitionExtra_  IndexOptions=Index vector (dialog)  Indices=1  OutputSizes=1
  Data Store Read92 : DataStoreRead  DataStoreName=oProp  DataStoreElements=oProp.oMot_.oParam_.fHardwareDelayCurrentAcquisition_  IndexOptions=Index vector (dialog)  Indices=1  OutputSizes=1
  Data Store Read93 : DataStoreRead  DataStoreName=oProp  DataStoreElements=oProp.oMot_.oParam_.fHardwareDelayControlLoopFraction_  IndexOptions=Index vector (dialog)  Indices=1  OutputSizes=1
  Data Store Write36 : DataStoreWrite  DataStoreName=oProp  DataStoreElements=oProp.oMot_.oState_.oRampDataFluxMasterAngleOffset_.fSetpoint_  IndexOptions=Index vector (dialog)  Indices=1  OutputSizes=1
  Data Store Write4 : DataStoreWrite  DataStoreName=oProp  DataStoreElements=oProp.oMot_.oOut_.fUphFilterAmplitudeRatio_  IndexOptions=Index vector (dialog)  Indices=1  OutputSizes=1
  Data Store Write43 : DataStoreWrite  DataStoreName=oProp  DataStoreElements=oProp.oMot_.oOut_.fUphFilterDelayAngleRad_  IndexOptions=Index vector (dialog)  Indices=1  OutputSizes=1
  Data Store Write8 : DataStoreWrite  DataStoreName=oProp  DataStoreElements=oProp.oMot_.oState_.fOmegaRel_  IndexOptions=Index vector (dialog)  Indices=1  OutputSizes=1
  Gain7 : Gain  Gain=1.414213562
  Product{,5..6,12..13} (5 alike) : Product
  Product1 : Product  OutDataTypeStr=single
  Saturation : Saturate  UpperLimit=inf  LowerLimit=0.3
  Saturation1 : Saturate  UpperLimit=pi/2  LowerLimit=-inf
  Sign : Signum
  Sign1 : Signum
  Variant Subsystem : Subsystem  Variant=on
  fTemp1 : Fcn  Expr=1-u
  wires:
  Sign1/1 -> Product6/1
  Product5/1 -> Product6/2  "fHardwareDelayAngleRad"
  Add5/1 -> Product5/2
  Abs4/1 -> Product5/1
  Product12/1 -> Add4/2
  Data Store Read26/1 -> Sign/1, Abs4/1, Abs/1  "fOmegaE"
  Add4/1 -> Saturation1/1
  Abs1/1 -> Product/1
  fTemp1/1 -> Atan3/2
  Data Store Read33/1 -> Product12/2
  Product13/1 -> Add5/2
  Saturation/1 -> Data Store Write4/1  "fUphFilterAmplitudeRatio_"
  Variant Subsystem/1(Out1) -> Product1/1, Data Store Write8/1, Product1/2, Gain7/1
  Abs/1 -> Variant Subsystem/1(In1), Product12/1
  Sign/1 -> Product/2, Sign1/1
  Data Store Read14/1 -> Product13/2
  Product/1 -> Data Store Write43/1  "fUphFilterDelayAngleRad_"
  Saturation1/1 -> Abs1/1
  Data Store Read93/1 -> Product13/1
  Atan3/1 -> Add4/1
  Gain7/1 -> Atan3/1
  Product6/1 -> Data Store Write36/1
  Data Store Read92/1 -> Add5/1
  Product1/1 -> AmplitudeRatio/1, fTemp1/1
  AmplitudeRatio/1 -> Saturation/1
